simulink model "my_foc9"  (R2024b)
settings: Solver=FixedStepDiscrete  StartTime=0.0  StopTime=2  FixedStep=0.000001  RelTol=1e-3  EnableMultiTasking=on
InitFcn:
  | D_PI_P = 2.19
  | D_PI_I = 1650.0
  | D_PI_UP_LIMIT = 3.0
  | D_PI_LOW_LIMIT = -3.0
  | D_PI_KB = 15
  | 
  | Q_PI_P = 2.19
  | Q_PI_I = 1650.0
  | Q_PI_UP_LIMIT = 3.0
  | Q_PI_LOW_LIMIT = -3.0
  | Q_PI_KB = 15
  | 
  | R = 0.6
  | Ld = 0.000558
  | Lq = 0.000558
  | Pn = 4
  | flux = 0.00572
  | PI = 3.1415926
  | Ts = 0.0001
values from neighbouring files (symbols this model uses):
  D_Upper_lower : value not decoded    [My_PID_parameter.sldd]
  OUT_limits : value not decoded    [My_PID_parameter.sldd]
  Q_KI = 1650.0    [My_PID_parameter.sldd]
  Q_KP = 2.19    [My_PID_parameter.sldd]
  SPEED_PI_I = 3.0    [My_PID_parameter.sldd]
  SPEED_PI_KB = 0.15    [My_PID_parameter.sldd]
  SPEED_PI_LOW_LIMIT = -5.0    [My_PID_parameter.sldd]
  SPEED_PI_P = 0.02    [My_PID_parameter.sldd]
  SPEED_PI_UP_LIMIT = 5.0    [My_PID_parameter.sldd]
undefined symbols (not defined in the file or in its folder): DiscIntNeverNeededParam
libraries: slpidlib x2, spsDCVoltageSourceLib x1, spsGroundLib x1, spsPermanentMagnetSynchronousMachineLib x1, simulink x1, spsThreePhaseVIMeasurementLib x1, spsUniversalBridgeLib x1, spspowerguiLib x1
settings Model: DataDictionary=My_PID_parameter.sldd  EnableAccessToBaseWorkspace=off  Creator=HRT  LastModifiedBy=12894
settings SolverCC: AlgebraicLoopSolver=TrustRegion
settings DataIOCC: ReturnWorkspaceOutputs=off
settings OptimizationCC: DefaultParameterBehavior=Inlined  UseDivisionForNetSlopeComputation=on  UseFloatMulNetSlope=on  DefaultUnderspecifiedDataType=single  InlineInvariantSignals=on  PassReuseOutputArgsAs=Individual arguments  ZeroExternalMemoryAtStartup=off  ZeroInternalMemoryAtStartup=off  NoFixptDivByZeroProtection=on  EfficientFloat2IntCast=on  LifeSpan=1  MaxStackSize=64  OptimizeBlockOrder=speed  DifferentSizesBufferReuse=on  EfficientTunableParamExpr=on
settings DebuggingCC: ParameterTunabilityLossMsg=error  UnconnectedInputMsg=warning  UnconnectedOutputMsg=warning  UnconnectedLineMsg=warning  ArithmeticOperatorsInVariantConditions=warning
settings HardwareCC: ProdBitPerPointer=32  ProdBitPerSizeT=32  ProdBitPerPtrDiffT=32  ProdLargestAtomicInteger=Long  ProdLargestAtomicFloat=Double  ProdWordSize=32  ProdLongLongMode=on  ProdHWDeviceType=ARM Compatible->ARM Cortex
settings ModelReferenceCC: EnableRefExpFcnMdlSchedulingChecks=on
settings SFSimCC: MATLABDynamicMemAlloc=off  CustomCodeUndefinedFunction=UseInterfaceOnly
settings RTWCC: Description=Embedded Coder  SystemTargetFile=ert.tlc  HardwareBoard=STM32F4-Discovery  TemplateMakefile=ert_default_tmf  GenerateReport=on  Toolchain=GNU Tools for ARM Embedded Processors  IncludeHyperlinkInReport=on  LaunchReport=on  GenerateTraceInfo=on  GenerateTraceReport=on  GenerateTraceReportSl=on  GenerateTraceReportSf=on  GenerateTraceReportEml=on  GenerateCodeMetricsReport=on  GPUComputeCapability=3.5
settings CodeAppCC: ForceParamTrailComments=on  IgnoreCustomStorageClasses=off  OperatorAnnotations=on  SimulinkDataObjDesc=on  SFDataObjDesc=on  CustomSymbolStrGlobalVar=rt$N$M  CustomSymbolStrType=$N$M  CustomSymbolStrFcn=$N$M$F  CustomSymbolStrMacro=$N$M  InsertBlockDesc=on
settings ERTTargetCC: CodeReplacementLibrary=ARM Cortex-M (CMSIS)  IncludeMdlTerminateFcn=off  CombineSignalStateStructs=on  SupportComplex=off  SupportNonInlinedSFcns=on  ERTFilePackagingFormat=CompactWithDataFile  DynamicArrayContainerType=coder::array

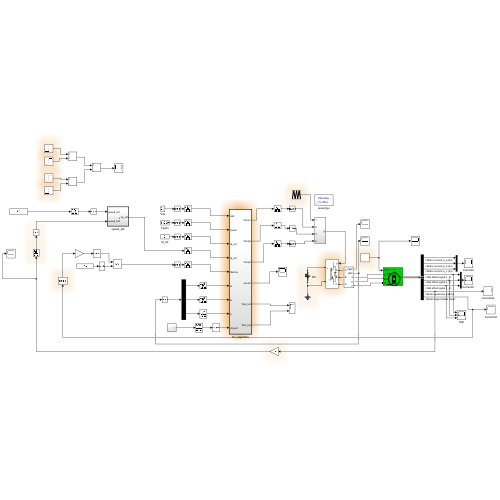
[thumbnail: Simulink's stored preview of the top-level diagram]
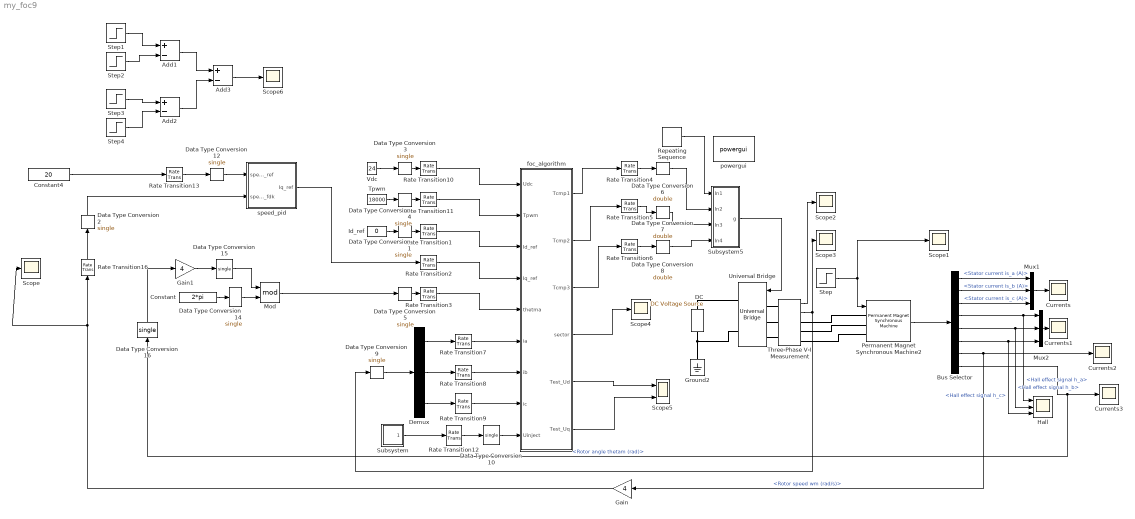
== system my_foc9 ==
  Add1 : Sum  Inputs=+-
  Add2 : Sum  Inputs=+-
  Add3 : Sum  Inputs=+-
  Bus Selector : BusSelector  OutputSignals=Stator current is_a (A),Stator current is_b (A),Stator current is_c (A),Hall effect signal h_a,Hall effect signal h_b,Hall effect signal h_c,Rotor speed wm (rad/s),Rotor angle thetam (rad)
  Constant : Constant  Value=2*pi
  Constant4 : Constant  Value=20  OutDataTypeStr=single
  Currents{,1..3} (4 alike) : Scope
  "DC " : spsDCVoltageSourceLib/DC Voltage Source  Amplitude=24  Measurements=None
  Data Type Conversion{1..5,9..10,12,14..16} (11 alike) : DataTypeConversion  OutDataTypeStr=single  SaturateOnIntegerOverflow=off  RndMeth=Floor
  Data Type Conversion6 : DataTypeConversion  OutDataTypeStr=double  SaturateOnIntegerOverflow=off  RndMeth=Floor
  Data Type Conversion7 : DataTypeConversion  OutDataTypeStr=double  SaturateOnIntegerOverflow=off  RndMeth=Floor
  Data Type Conversion8 : DataTypeConversion  OutDataTypeStr=double  SaturateOnIntegerOverflow=off  RndMeth=Floor
  Demux : Demux  Outputs=3
  Gain : Gain  Gain=4
  Gain1 : Gain  Gain=4
  Ground2 : spsGroundLib/Ground  LConnTagsString=a
  Hall : Scope  NumInputPorts=3
  Id_ref : Constant  Value=0
  Mod : Math  Operator=mod  SignedPower=on
  Mux1 : Mux  Inputs=3
  Mux2 : Mux  Inputs=3
  Permanent Magnet Synchronous Machine2 : spsPermanentMagnetSynchronousMachineLib/Permanent Magnet Synchronous Machine  NbPhases=3  FluxDistribution=Sinusoidal  RotorType=Round  MechanicalLoad=Torque Tm  PresetModel=No  ShowDetailedParameters=on  MeasurementBus=off  Resistance=0.6  Inductance=8.5e-3  dqInductances=[8.5e-3, 8.5e-3]  La=5.58e-4  MachineConstant=Flux linkage established by magnets (V.s)  Flux=0.00572  VoltageCst=4.15  TorqueCst=0.03432  Flat=120  Mechanical=[1.1e-5,1e-4,4,0.02]  PolePairs=4  InitialConditions=[0,0, 0,0]  InitialConditions5ph=[0 0 0 0 0 0]  RefAngle=Aligned with phase A axis (original Park)  IterativeDiscreteModel=Trapezoidal non iterative  TsBlock=-1  TsPowergui=0
  Rate Transition{1..13,16} (14 alike) : RateTransition
  Repeating Sequence : simulink/Sources/Repeating Sequence  rep_seq_t=[0 0.0001 0.0002]  rep_seq_y=[0 9000 0]
  Scope{,1..4,6} (6 alike) : Scope
  Scope5 : Scope  NumInputPorts=2
  Step : Step  Time=0  After=0  SampleTime=0
  Step1 : Step  Time=0.1  After=2  SampleTime=0
  Step2 : Step  Time=0.11  After=2  SampleTime=0
  Step3 : Step  Time=0.13  After=2  SampleTime=0
  Step4 : Step  Time=0.14  After=2  SampleTime=0
  Subsystem : Subsystem
  Subsystem5 : Subsystem
  Three-Phase V-I Measurement : spsThreePhaseVIMeasurementLib/Three-Phase V-I Measurement  VoltageMeasurement=phase-to-ground  SetLabelV=off  LabelV=Vabc  Vpu=off  VpuLL=off  CurrentMeasurement=yes  SetLabelI=off  LabelI=Iabc  Ipu=off  Pbase=100e6  Vbase=500e3  OutputType=Complex  PhasorSimulation=off  PSBequivalent=0
  Tpwm : Constant  Value=18000
  Universal Bridge : spsUniversalBridgeLib/Universal Bridge  Arms=3  SnubberResistance=1e5  SnubberCapacitance=inf  Device=IGBT / Diodes  Ron=1e-3  Lon=0  ForwardVoltages="[  0  0  ]"  ForwardVoltage=0  GTOparameters=[ 10e-6 , 20e-6 ]  IGBTparameters=[ 1e-6 , 2e-6 ]  Measurements=None  Measurements_2=None  converterType=Rectifier
  Vdc : Constant  Value=24
  foc_algorithm : Subsystem  TreatAsAtomicUnit=on  SystemSampleTime=0.0001
  powergui : spspowerguiLib/powergui  Priority=1  SimulationMode=Discrete  SampleTime=0.000001  frequency=60  Iterations=50  frequencyindice=0  Pbase=100e6  ErrMax=1e-4  UnitsV=kV  UnitsW=MW  buscounter=0  FunctionMessages=off  echomessages=off  EnableUseOfTLC=off  CurrentSourceSwitches=off  DisableSnubberDevices=off  DisableRonSwitches=off  DisableVfSwitches=off  DisplayEquations=off  AutomaticDiscreteSolvers=off  SolverType=Tustin/Backward Euler (TBE)  Interpol=off  ExternalGateDelay=off  methode=off  Ts=100  x0status=blocks  SPID=off  SwTol=0  HookPort=off  NonlinearTolerance=1e-4  nMaxIteration=100  ContinueOnMaxIteration=off  RestoreLinks=warning  ResistiveCurrentMeasurement=off  Frange=[0:2:500]  Ylog=off  Xlog=on  ShowGrid=off  save=off  variable=ZData  structure=0  ZoomFFT=off  StartTime=0.0  cycles=1  DisplayStyle=1  fundamental=60  FreqAxis=off  MaxFrequency=1000  frequencyindicesteady=1  RmsSteady=1  display=off
  speed_pid : Subsystem  TreatAsAtomicUnit=on  SystemSampleTime=0.001
  wires:
  Mux2/1 -> Currents1/1
  Rate Transition6/1 -> Data Type Conversion8/1
  Rate Transition10/1 -> foc_algorithm/1(Udc)
  Vdc/1 -> Data Type Conversion3/1
  Data Type Conversion8/1 -> Subsystem5/4(In4)
  Bus Selector/4 -> Hall/1, Mux2/1  "<Hall effect signal h_a>"
  Id_ref/1 -> Data Type Conversion1/1
  Rate Transition2/1 -> foc_algorithm/4(Iq_ref)
  Rate Transition3/1 -> foc_algorithm/5(thetma)
  Mux1/1 -> Currents/1
  Three-Phase V-I Measurement/1 -> Scope2/1
  Data Type Conversion1/1 -> Rate Transition1/1
  Bus Selector/6 -> Mux2/3, Hall/3  "<Hall effect signal h_c>"
  Bus Selector/2 -> Mux1/2  "<Stator current is_b (A)>"
  Bus Selector/7 -> Gain/1, Currents2/1  "<Rotor speed wm (rad/s)>"
  Rate Transition5/1 -> Data Type Conversion7/1
  Rate Transition1/1 -> foc_algorithm/3(Id_ref)
  Data Type Conversion7/1 -> Subsystem5/3(In3)
  Repeating Sequence/1 -> Subsystem5/1(In1)
  foc_algorithm/1(Tcmp1) -> Rate Transition4/1
  Bus Selector/5 -> Mux2/2, Hall/2  "<Hall effect signal h_b>"
  foc_algorithm/3(Tcmp3) -> Rate Transition6/1
  Data Type Conversion5/1 -> Rate Transition3/1
  Rate Transition11/1 -> foc_algorithm/2(Tpwm)
  Bus Selector/3 -> Mux1/3  "<Stator current is_c (A)>"
  foc_algorithm/2(Tcmp2) -> Rate Transition5/1
  Data Type Conversion4/1 -> Rate Transition11/1
  Rate Transition4/1 -> Data Type Conversion6/1
  Data Type Conversion3/1 -> Rate Transition10/1
  Tpwm/1 -> Data Type Conversion4/1
  Bus Selector/8 -> Data Type Conversion16/1, Currents3/1  "<Rotor angle thetam (rad)>"
  Data Type Conversion6/1 -> Subsystem5/2(In2)
  Subsystem5/1(g) -> Universal Bridge/1
  speed_pid/1(Iq_ref) -> Rate Transition2/1
  Bus Selector/1 -> Mux1/1  "<Stator current is_a (A)>"
  foc_algorithm/4(sector) -> Scope4/1
  Demux/3 -> Rate Transition9/1
  Three-Phase V-I Measurement/2 -> Scope3/1, Data Type Conversion9/1
  Demux/2 -> Rate Transition8/1
  Demux/1 -> Rate Transition7/1
  Rate Transition7/1 -> foc_algorithm/6(ia)
  Rate Transition8/1 -> foc_algorithm/7(ib)
  Rate Transition9/1 -> foc_algorithm/8(ic)
  Data Type Conversion9/1 -> Demux/1
  Step/1 -> Permanent Magnet Synchronous Machine2/1, Scope1/1
  foc_algorithm/5(Test_Ud) -> Scope5/1
  foc_algorithm/6(Test_Uq) -> Scope5/2
  Gain1/1 -> Data Type Conversion15/1
  Rate Transition13/1 -> Data Type Conversion12/1
  Constant/1 -> Data Type Conversion14/1
  Data Type Conversion14/1 -> Mod/2
  Data Type Conversion16/1 -> Gain1/1
  Permanent Magnet Synchronous Machine2/1 -> Bus Selector/1
  Data Type Conversion15/1 -> Mod/1
  Constant4/1 -> Rate Transition13/1
  Rate Transition16/1 -> Data Type Conversion2/1
  Data Type Conversion2/1 -> speed_pid/2(speed_fdk)
  Gain/1 -> Scope/1, Rate Transition16/1
  Mod/1 -> Data Type Conversion5/1
  Step1/1 -> Add1/1
  Step2/1 -> Add1/2
  Step3/1 -> Add2/1
  Step4/1 -> Add2/2
  Add1/1 -> Add3/1
  Add2/1 -> Add3/2
  Add3/1 -> Scope6/1
  Subsystem/1(Out1) -> Rate Transition12/1
  Rate Transition12/1 -> Data Type Conversion10/1
  Data Type Conversion10/1 -> foc_algorithm/9("Uinject ")
  Data Type Conversion12/1 -> speed_pid/1(speed_ref)
  connections:
  Ground2/LConn1 -- Universal Bridge/RConn2 -- "DC "/LConn1
  "DC "/RConn1 -- Universal Bridge/RConn1
  Universal Bridge/LConn2 -- Three-Phase V-I Measurement/LConn2
  Universal Bridge/LConn1 -- Three-Phase V-I Measurement/LConn1
  Permanent Magnet Synchronous Machine2/LConn3 -- Three-Phase V-I Measurement/RConn3
  Universal Bridge/LConn3 -- Three-Phase V-I Measurement/LConn3
  Permanent Magnet Synchronous Machine2/LConn2 -- Three-Phase V-I Measurement/RConn2
  Permanent Magnet Synchronous Machine2/LConn1 -- Three-Phase V-I Measurement/RConn1

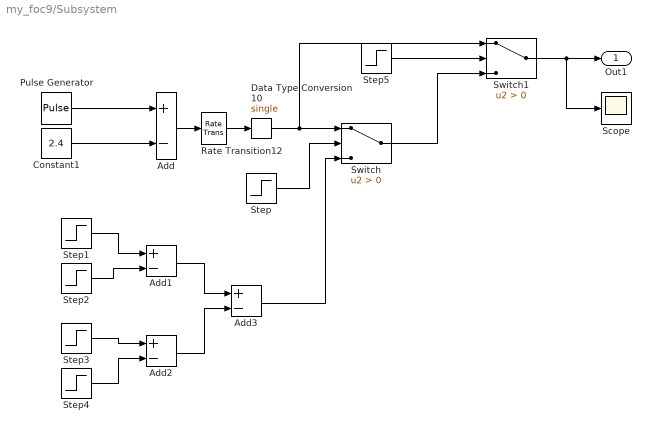
== system my_foc9/Subsystem ==
  Add{,1..3} (4 alike) : Sum  Inputs=+-
  Constant1 : Constant  Value=2.4
  Data Type Conversion10 : DataTypeConversion  OutDataTypeStr=single  SaturateOnIntegerOverflow=off  RndMeth=Floor
  Pulse Generator : DiscretePulseGenerator  PulseType=Time based  Amplitude=4.8  Period=0.0002  PulseWidth=50
  Rate Transition12 : RateTransition
  Scope : Scope
  Step : Step  Time=0.5  Before=1  After=0  SampleTime=0
  Step1 : Step  Time=0.6  After=2  SampleTime=0
  Step2 : Step  Time=0.7  After=2  SampleTime=0
  Step3 : Step  Time=0.8  After=2  SampleTime=0
  Step4 : Step  Time=0.9  After=2  SampleTime=0
  Step5 : Step  After=2  SampleTime=0
  Switch : Switch  Criteria=u2 > Threshold  SaturateOnIntegerOverflow=off  InputSameDT=off
  Switch1 : Switch  Criteria=u2 > Threshold  SaturateOnIntegerOverflow=off  InputSameDT=off
  Out1 : Outport  VectorParamsAs1DForOutWhenUnconnected=off
  wires:
  Constant1/1 -> Add/2
  Rate Transition12/1 -> Data Type Conversion10/1
  Pulse Generator/1 -> Add/1
  Add/1 -> Rate Transition12/1
  Switch/1 -> Switch1/3
  Step3/1 -> Add2/1
  Step1/1 -> Add1/1
  Add2/1 -> Add3/2
  Add1/1 -> Add3/1
  Step2/1 -> Add1/2
  Step4/1 -> Add2/2
  Data Type Conversion10/1 -> Switch1/1, Switch/1
  Step/1 -> Switch/2
  Step5/1 -> Switch1/2
  Switch1/1 -> Scope/1, Out1/1
  Add3/1 -> Switch/3

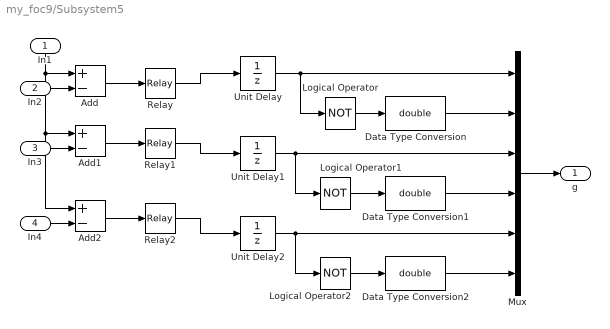
== system my_foc9/Subsystem5 ==
  In1 : Inport
  In2 : Inport  Port=2
  In3 : Inport  Port=3
  In4 : Inport  Port=4
  Add : Sum  Inputs=+-
  Add1 : Sum  Inputs=+-
  Add2 : Sum  Inputs=+-
  Data Type Conversion : DataTypeConversion  OutDataTypeStr=double  SaturateOnIntegerOverflow=off  RndMeth=Floor
  Data Type Conversion1 : DataTypeConversion  OutDataTypeStr=double  SaturateOnIntegerOverflow=off  RndMeth=Floor
  Data Type Conversion2 : DataTypeConversion  OutDataTypeStr=double  SaturateOnIntegerOverflow=off  RndMeth=Floor
  Logical Operator : Logic  Operator=NOT  AllPortsSameDT=off  OutDataTypeStr=boolean
  Logical Operator1 : Logic  Operator=NOT  AllPortsSameDT=off  OutDataTypeStr=boolean
  Logical Operator2 : Logic  Operator=NOT  AllPortsSameDT=off  OutDataTypeStr=boolean
  Mux : Mux  Inputs=6
  Relay : Relay  OffSwitchValue=-eps
  Relay1 : Relay  OffSwitchValue=-eps
  Relay2 : Relay  OffSwitchValue=-eps
  Unit Delay : UnitDelay  SampleTime=-1  HasFrameUpgradeWarning=on
  Unit Delay1 : UnitDelay  SampleTime=-1  HasFrameUpgradeWarning=on
  Unit Delay2 : UnitDelay  SampleTime=-1  HasFrameUpgradeWarning=on
  g : Outport  VectorParamsAs1DForOutWhenUnconnected=off
  wires:
  In4/1 -> Add2/2
  In3/1 -> Add1/2
  In2/1 -> Add/2
  Relay2/1 -> Unit Delay2/1
  Relay1/1 -> Unit Delay1/1
  Relay/1 -> Unit Delay/1
  Unit Delay2/1 -> Mux/5, Logical Operator2/1
  Unit Delay1/1 -> Mux/3, Logical Operator1/1
  Unit Delay/1 -> Logical Operator/1, Mux/1
  Mux/1 -> g/1
  Data Type Conversion/1 -> Mux/2
  Data Type Conversion1/1 -> Mux/4
  Data Type Conversion2/1 -> Mux/6
  Logical Operator2/1 -> Data Type Conversion2/1
  Logical Operator1/1 -> Data Type Conversion1/1
  Logical Operator/1 -> Data Type Conversion/1
  Add1/1 -> Relay1/1
  Add2/1 -> Relay2/1
  Add/1 -> Relay/1
  In1/1 -> Add/1, Add2/1, Add1/1

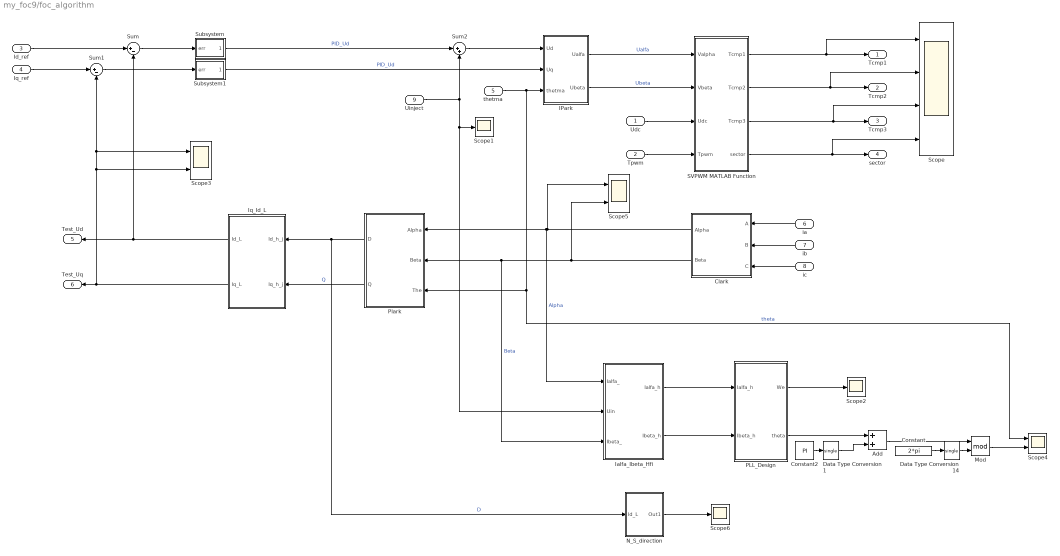
== system my_foc9/foc_algorithm ==
  Udc : Inport
  Tpwm : Inport  Port=2
  Id_ref : Inport  Port=3
  Iq_ref : Inport  Port=4
  thetma : Inport  Port=5
  ia : Inport  Port=6
  ib : Inport  Port=7
  ic : Inport  Port=8
  "Uinject " : Inport  Port=9
  Add : Sum
  Clark : Subsystem
  Constant : Constant  Value=2*pi
  Constant2 : Constant  Value=PI
  Data Type Conversion1 : DataTypeConversion  OutDataTypeStr=single  SaturateOnIntegerOverflow=off  RndMeth=Floor
  Data Type Conversion14 : DataTypeConversion  OutDataTypeStr=single  SaturateOnIntegerOverflow=off  RndMeth=Floor
  IPark : Subsystem
  "Ialfa_Ibeta_Hfi " : Subsystem  TreatAsAtomicUnit=on  SystemSampleTime=Ts
  Iq_Id_L : Subsystem
  Mod : Math  Operator=mod  SignedPower=on
  N_S_direction : Subsystem  TreatAsAtomicUnit=on  SystemSampleTime=Ts
  PLL_Design : Subsystem  TreatAsAtomicUnit=on  SystemSampleTime=Ts
  Plark : Subsystem
  SVPWM MATLAB Function : MATLAB Function  TreatAsAtomicUnit=on
  Scope : Scope  NumInputPorts=4
  Scope1 : Scope
  Scope2 : Scope
  Scope3 : Scope  NumInputPorts=2
  Scope4 : Scope  NumInputPorts=2
  Scope5 : Scope  NumInputPorts=2
  Scope6 : Scope
  Subsystem : Subsystem  mask(my_pi){kp=Q_KP, ki=Q_KI, Intergral_Limits=D_Upper_lower, Output_Limits=OUT_limits, init=0, TS=0.0001}
      mask prompts: kp "Proportional gain(kp):"; ki "Intergral gain(ki):"; Intergral_Limits "Intergral limits:[Upper Lowers]"; Output_Limits "Output limits:[Upper Lower]"; init "Output init value:"; TS "Sample time:"
      mask init:
      | Intergral_upper =Intergral_Limits(1);
      | Intergral_lower = Intergral_Limits(2);
      | Out_upper       = Output_Limits(1);
      | Out_lower       = Output_Limits(2);
      mask Display: disp('PI')
  Subsystem1 : Subsystem  mask(my_pi){kp=Q_KP, ki=Q_KI, Intergral_Limits=D_Upper_lower, Output_Limits=OUT_limits, init=0, TS=0.0001}
      mask prompts: kp "Proportional gain(kp):"; ki "Intergral gain(ki):"; Intergral_Limits "Intergral limits:[Upper Lowers]"; Output_Limits "Output limits:[Upper Lower]"; init "Output init value:"; TS "Sample time:"
      mask init:
      | Intergral_upper =Intergral_Limits(1);
      | Intergral_lower = Intergral_Limits(2);
      | Out_upper       = Output_Limits(1);
      | Out_lower       = Output_Limits(2);
      mask Display: disp('PI')
  Sum : Sum  Inputs=|+-
  Sum1 : Sum  Inputs=|+-
  Sum2 : Sum  Inputs=|++
  Tcmp1 : Outport  VectorParamsAs1DForOutWhenUnconnected=off
  Tcmp2 : Outport  Port=2  VectorParamsAs1DForOutWhenUnconnected=off
  Tcmp3 : Outport  Port=3  VectorParamsAs1DForOutWhenUnconnected=off
  sector : Outport  Port=4  VectorParamsAs1DForOutWhenUnconnected=off
  Test_Ud : Outport  Port=5  VectorParamsAs1DForOutWhenUnconnected=off
  Test_Uq : Outport  Port=6  VectorParamsAs1DForOutWhenUnconnected=off
  wires:
  IPark/1(Ualfa) -> SVPWM MATLAB Function/1(Valpha)  "Ualfa"
  IPark/2(Ubeta) -> SVPWM MATLAB Function/2(Vbeta)  "Ubeta"
  Udc/1 -> SVPWM MATLAB Function/3(Udc)
  Tpwm/1 -> SVPWM MATLAB Function/4(Tpwm)
  SVPWM MATLAB Function/1(Tcmp1) -> Scope/1, Tcmp1/1
  SVPWM MATLAB Function/2(Tcmp2) -> Scope/2, Tcmp2/1
  SVPWM MATLAB Function/3(Tcmp3) -> Scope/3, Tcmp3/1
  thetma/1 -> Scope4/1, Plark/3(The), IPark/3(thetma)  "theta"
  SVPWM MATLAB Function/4(sector) -> Scope/4, sector/1
  Clark/1(Alpha) -> "Ialfa_Ibeta_Hfi "/1(Ialfa_), Plark/1(Alpha), Scope5/1  "Alpha"
  Clark/2(Beta) -> Scope5/2, "Ialfa_Ibeta_Hfi "/3(Ibeta_), Plark/2(Beta)  "Beta"
  Sum/1 -> Subsystem/1("err ")
  Sum1/1 -> Subsystem1/1("err ")
  Plark/1(D) -> N_S_direction/1(Id_L), Iq_Id_L/1(Id_h_j)  "D"
  Plark/2(Q) -> Iq_Id_L/2(Iq_h_j)  "Q"
  ia/1 -> Clark/1(A)
  ib/1 -> Clark/2(B)
  ic/1 -> Clark/3(C)
  Iq_ref/1 -> Sum1/1
  Id_ref/1 -> Sum/1
  "Uinject "/1 -> "Ialfa_Ibeta_Hfi "/2("Uin "), Scope1/1, Sum2/2
  "Ialfa_Ibeta_Hfi "/2(Ibeta_h) -> PLL_Design/2("Ibeta_h ")
  "Ialfa_Ibeta_Hfi "/1("Ialfa_h ") -> PLL_Design/1(Ialfa_h)
  PLL_Design/1("We ") -> Scope2/1
  Sum2/1 -> IPark/1(Ud)
  Subsystem/1(Out1) -> Sum2/1  "PID_Ud"
  Subsystem1/1(Out1) -> IPark/2(Uq)  "PID_Ud"
  Iq_Id_L/2(Iq_L) -> Scope3/2, Sum1/2, Scope3/1, Test_Uq/1
  Iq_Id_L/1(Id_L) -> Sum/2, Test_Ud/1
  Data Type Conversion14/1 -> Mod/2
  Constant/1 -> Data Type Conversion14/1
  Mod/1 -> Scope4/2
  PLL_Design/2(theta) -> Add/1
  Add/1 -> Mod/1
  Constant2/1 -> Data Type Conversion1/1
  Data Type Conversion1/1 -> Add/2
  N_S_direction/1(Out1) -> Scope6/1

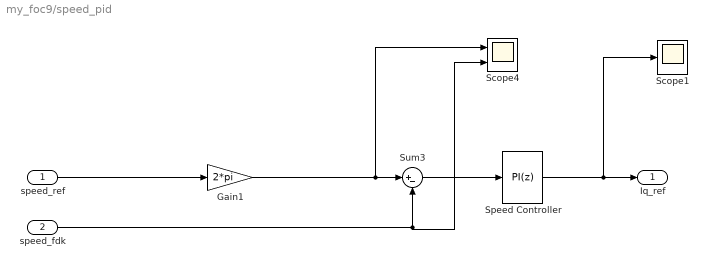
== system my_foc9/speed_pid ==
  speed_ref : Inport
  speed_fdk : Inport  Port=2
  Gain1 : Gain  Gain=2*pi  OutDataTypeStr=single
  Scope1 : Scope
  Scope4 : Scope  NumInputPorts=2
  Speed Controller : slpidlib/PID Controller  Controller=PI  Form=Ideal  TimeDomain=Discrete-time  UseExternalTs=off  SampleTime=-1  IntegratorMethod=Forward Euler  FilterMethod=Forward Euler  ControllerParametersSource=internal  P=SPEED_PI_P  I=SPEED_PI_I  UseKiTs=off  D=0.0005  UseExternalDerivativeSource=off  N=100  UseFilter=on  TunerSelectOption=Transfer Function Based (PID Tuner App)  InitialConditionSource=internal  InitialConditionForIntegrator=0  InitialConditionForFilter=0  DifferentiatorICPrevScaledInput=0  ExternalReset=none  TrackingMode=off  Kt=1  LimitOutput=on  SatLimitsSource=internal  UpperSaturationLimit=SPEED_PI_UP_LIMIT  LowerSaturationLimit=SPEED_PI_LOW_LIMIT  LinearizeAsGain=off  AntiWindupMode=back-calculation  Kb=SPEED_PI_KB  LimitIntegrator=off  UpperIntegratorSaturationLimit=inf  LowerIntegratorSaturationLimit=-inf  PGainOutDataTypeStr=single  PProdOutDataTypeStr=single  POutMin=[]  POutMax=[]  IGainOutDataTypeStr=single  IProdOutDataTypeStr=single  IOutMin=[]  IOutMax=[]  DOutMin=[]  DOutMax=[]  NOutMin=[]  NOutMax=[]  SumOutDataTypeStr=single  SumOutMin=[]  SumOutMax=[]  SaturationOutDataTypeStr=single  SaturationOutMin=[]  SaturationOutMax=[]  PParamDataTypeStr=single  PParamMin=[]  PParamMax=[]  IParamDataTypeStr=single  IParamMin=[]  IParamMax=[]  DParamMin=[]  DParamMax=[]  NParamMin=[]  NParamMax=[]  KbParamDataTypeStr=single  KbParamMin=[]  KbParamMax=[]  KtParamMin=[]  KtParamMax=[]  KbOutDataTypeStr=single  KbOutMin=[]  KbOutMax=[]  KtOutMin=[]  KtOutMax=[]  IntegratorOutDataTypeStr=single  IntegratorOutMin=[]  IntegratorOutMax=[]  FilterOutMin=[]  FilterOutMax=[]  SumI1OutDataTypeStr=single  SumI1OutMin=[]  SumI1OutMax=[]  SumI2OutDataTypeStr=single  SumI2OutMin=[]  SumI2OutMax=[]  SumI3OutMin=[]  SumI3OutMax=[]  SumI4OutMin=[]  SumI4OutMax=[]  SumDOutMin=[]  SumDOutMax=[]  SumAccumDataTypeStr=single  SumI1AccumDataTypeStr=single  SumI2AccumDataTypeStr=single  DifferentiatorOutMin=[]  DifferentiatorOutMax=[]  FilterDiffOutCoefMin=[]  FilterDiffOutCoefMax=[]  ReciprocalOutMin=[]  ReciprocalOutMax=[]  SumDenOutMin=[]  SumDenOutMax=[]  SumNumOutMin=[]  SumNumOutMax=[]  DivideOutMin=[]  DivideOutMax=[]  UdiffTsProdOutMin=[]  UdiffTsProdOutMax=[]  NTsProdOutMin=[]  NTsProdOutMax=[]  UintegralTsProdOutMin=[]  UintegralTsProdOutMax=[]  UngainTsProdOutMin=[]  UngainTsProdOutMax=[]  ClampingZeroOutDataTypeStr=Inherit: Inherit via back propagation  ClampingZeroOutMin=[]  ClampingZeroOutMax=[]  FilterDenConstantOutDataTypeStr=Inherit: Inherit via back propagation  FilterDenConstantOutMin=[]  FilterDenConstantOutMax=[]  PCopyOutDataTypeStr=Inherit: Inherit via back propagation  PCopyOutMin=[]  PCopyOutMax=[]  NCopyOutDataTypeStr=Inherit: Inherit via back propagation  NCopyOutMin=[]  NCopyOutMax=[]  IntegratorContinuousStateAttributes=''  IntegratorStateIdentifier=si  IntegratorStateMustResolveToSignalObject=off  IntegratorRTWStateStorageClass=Auto  FilterContinuousStateAttributes=''  FilterStateMustResolveToSignalObject=off  FilterRTWStateStorageClass=Auto  ParallelPVariant=Passthrough  IdealPVariant=InternalParameters  IVariant=InternalParameters  DVariant=Disabled  IntegratorVariant=Discrete  SatVariant=Enabled  AWVariant=BackCalculation  PCopyVariant=Disabled  TRVariant=Disabled  FdbkBlocksVariant=Forward  IdealPFdbkVariant=Disabled  SatFdbkVariant=Disabled  DerivativeFilterVariant=Disabled  NVariant=Disabled  NCopyVariant=Disabled_SignalSpec  FilterICVariant=Disabled  IntegratorICVariant=InternalICs  ExternalResetVariant=Disabled  TRSumVariant=Passthrough  SumFdbkVariant=Disabled  SumVariant=Sum_PI  TsampFilterVariant=InternalTs  TsampNgainVariant=Passthrough  TsampIntegralVariant=Disabled_SignalSpec  ExternalSaturationOutDataTypeStr=Inherit: Same as second input  DerivativeSourceVariant=Disabled  PreIntVariant=InternalPreInt
  Sum3 : Sum  Inputs=|+-  InputSameDT=on
  Iq_ref : Outport  VectorParamsAs1DForOutWhenUnconnected=off
  wires:
  Sum3/1 -> Speed Controller/1
  speed_ref/1 -> Gain1/1
  Speed Controller/1 -> Scope1/1, Iq_ref/1
  speed_fdk/1 -> Scope4/2, Sum3/2
  Gain1/1 -> Sum3/1, Scope4/1

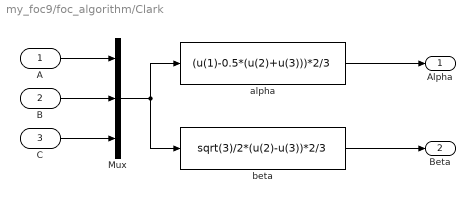
== system my_foc9/foc_algorithm/Clark ==
  A : Inport
  B : Inport  Port=2
  C : Inport  Port=3
  Mux : Mux  Inputs=3
  alpha : Fcn  Expr=(u(1)-0.5*(u(2)+u(3)))*2/3
  beta : Fcn  Expr=sqrt(3)/2*(u(2)-u(3))*2/3
  Alpha : Outport  VectorParamsAs1DForOutWhenUnconnected=off
  Beta : Outport  Port=2  VectorParamsAs1DForOutWhenUnconnected=off
  wires:
  alpha/1 -> Alpha/1
  B/1 -> Mux/2
  C/1 -> Mux/3
  A/1 -> Mux/1
  Mux/1 -> beta/1, alpha/1
  beta/1 -> Beta/1

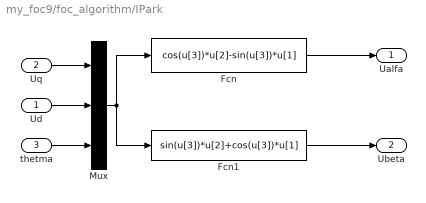
== system my_foc9/foc_algorithm/IPark ==
  Ud : Inport
  Uq : Inport  Port=2
  thetma : Inport  Port=3
  Fcn : Fcn  Expr=cos(u[3])*u[2]-sin(u[3])*u[1]
  Fcn1 : Fcn  Expr=sin(u[3])*u[2]+cos(u[3])*u[1]
  Mux : Mux  Inputs=3
  Ualfa : Outport  VectorParamsAs1DForOutWhenUnconnected=off
  Ubeta : Outport  Port=2  VectorParamsAs1DForOutWhenUnconnected=off
  wires:
  Uq/1 -> Mux/1
  Ud/1 -> Mux/2
  thetma/1 -> Mux/3
  Mux/1 -> Fcn/1, Fcn1/1
  Fcn/1 -> Ualfa/1
  Fcn1/1 -> Ubeta/1

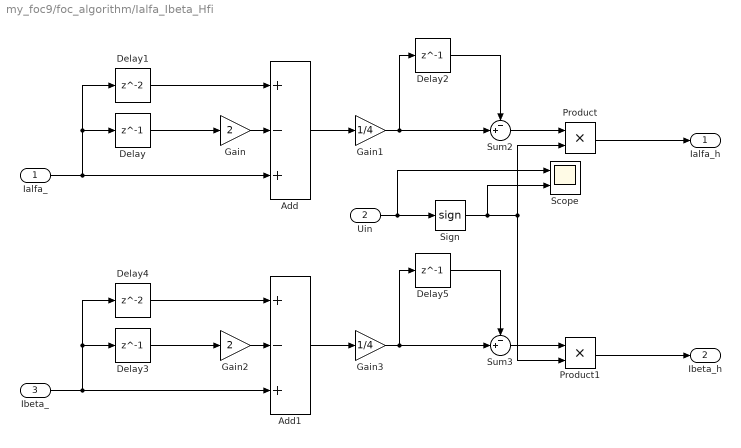
== system my_foc9/foc_algorithm/Ialfa_Ibeta_Hfi  ==
  Ialfa_ : Inport
  "Uin " : Inport  Port=2
  Ibeta_ : Inport  Port=3
  Add : Sum  Inputs=+-+
  Add1 : Sum  Inputs=+-+
  Delay{,2..3,5} (4 alike) : Delay  DelayLength=1  SampleTime=Ts
  Delay1 : Delay  SampleTime=Ts
  Delay4 : Delay  SampleTime=Ts
  Gain : Gain  Gain=2
  Gain1 : Gain  Gain=1/4
  Gain2 : Gain  Gain=2
  Gain3 : Gain  Gain=1/4
  Product : Product
  Product1 : Product
  Scope : Scope  NumInputPorts=2
  Sign : Signum
  Sum2 : Sum  Inputs=-+|
  Sum3 : Sum  Inputs=-+|
  "Ialfa_h " : Outport  VectorParamsAs1DForOutWhenUnconnected=off
  Ibeta_h : Outport  Port=2  VectorParamsAs1DForOutWhenUnconnected=off
  wires:
  Sign/1 -> Scope/2, Product/2, Product1/2
  Ialfa_/1 -> Delay1/1, Delay/1, Add/3
  "Uin "/1 -> Scope/1, Sign/1
  Gain3/1 -> Delay5/1, Sum3/2
  Ibeta_/1 -> Delay4/1, Delay3/1, Add1/3
  Gain/1 -> Add/2
  Gain1/1 -> Delay2/1, Sum2/2
  Delay1/1 -> Add/1
  Gain2/1 -> Add1/2
  Sum2/1 -> Product/1
  Add1/1 -> Gain3/1
  Sum3/1 -> Product1/1
  Product1/1 -> Ibeta_h/1
  Delay5/1 -> Sum3/1
  Delay3/1 -> Gain2/1
  Product/1 -> "Ialfa_h "/1
  Delay4/1 -> Add1/1
  Delay2/1 -> Sum2/1
  Delay/1 -> Gain/1
  Add/1 -> Gain1/1

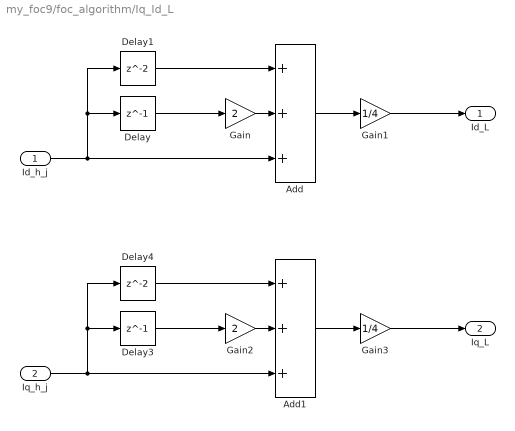
== system my_foc9/foc_algorithm/Iq_Id_L ==
  Id_h_j : Inport
  Iq_h_j : Inport  Port=2
  Add : Sum  Inputs=+++
  Add1 : Sum  Inputs=+++
  Delay : Delay  DelayLength=1  SampleTime=Ts
  Delay1 : Delay  SampleTime=Ts
  Delay3 : Delay  DelayLength=1  SampleTime=Ts
  Delay4 : Delay  SampleTime=Ts
  Gain : Gain  Gain=2
  Gain1 : Gain  Gain=1/4
  Gain2 : Gain  Gain=2
  Gain3 : Gain  Gain=1/4
  Id_L : Outport  VectorParamsAs1DForOutWhenUnconnected=off
  Iq_L : Outport  Port=2  VectorParamsAs1DForOutWhenUnconnected=off
  wires:
  Delay3/1 -> Gain2/1
  Iq_h_j/1 -> Delay4/1, Delay3/1, Add1/3
  Delay1/1 -> Add/1
  Gain/1 -> Add/2
  Gain2/1 -> Add1/2
  Delay4/1 -> Add1/1
  Add/1 -> Gain1/1
  Add1/1 -> Gain3/1
  Delay/1 -> Gain/1
  Id_h_j/1 -> Delay1/1, Delay/1, Add/3
  Gain1/1 -> Id_L/1
  Gain3/1 -> Iq_L/1

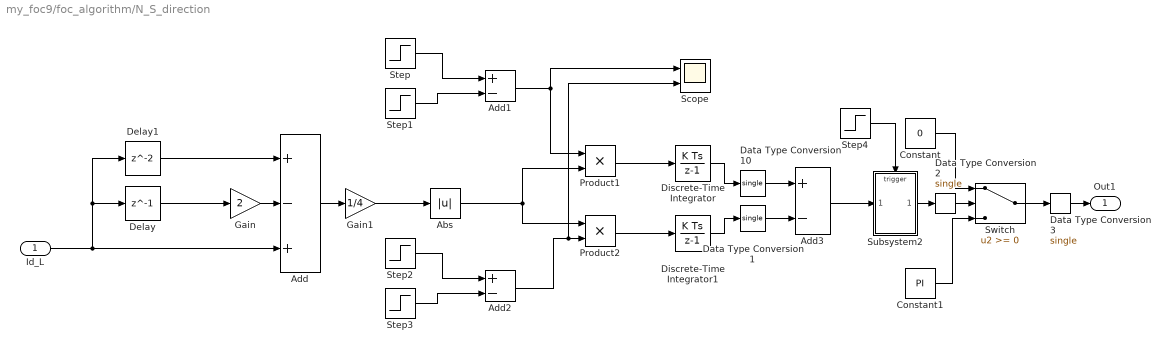
== system my_foc9/foc_algorithm/N_S_direction ==
  Id_L : Inport
  Abs : Abs  SaturateOnIntegerOverflow=off
  Add : Sum  Inputs=+-+
  Add1 : Sum  Inputs=+-
  Add2 : Sum  Inputs=+-
  Add3 : Sum  Inputs=+-
  Constant : Constant  Value=0
  Constant1 : Constant  Value=PI
  Data Type Conversion{1..3,10} (4 alike) : DataTypeConversion  OutDataTypeStr=single  SaturateOnIntegerOverflow=off  RndMeth=Floor
  Delay : Delay  DelayLength=1  SampleTime=Ts
  Delay1 : Delay  SampleTime=Ts
  Discrete-Time Integrator : DiscreteIntegrator  SampleTime=Ts  ICPrevOutput=DiscIntNeverNeededParam  ICPrevScaledInput=DiscIntNeverNeededParam
  Discrete-Time Integrator1 : DiscreteIntegrator  SampleTime=Ts  ICPrevOutput=DiscIntNeverNeededParam  ICPrevScaledInput=DiscIntNeverNeededParam
  Gain : Gain  Gain=2
  Gain1 : Gain  Gain=1/4
  Product1 : Product
  Product2 : Product
  Scope : Scope  NumInputPorts=2
  Step : Step  Time=0.6  After=2  SampleTime=Ts
  Step1 : Step  Time=0.7  After=2  SampleTime=Ts
  Step2 : Step  Time=0.8  After=2  SampleTime=Ts
  Step3 : Step  Time=0.9  After=2  SampleTime=Ts
  Step4 : Step  Time=0.16  SampleTime=Ts
  Subsystem2 : Subsystem
  Switch : Switch  SaturateOnIntegerOverflow=off  InputSameDT=off
  Out1 : Outport  VectorParamsAs1DForOutWhenUnconnected=off
  wires:
  Step4/1 -> Subsystem2/Trigger
  Switch/1 -> Data Type Conversion3/1
  Add2/1 -> Scope/2, Product2/2
  Step/1 -> Add1/1
  Product2/1 -> Discrete-Time Integrator1/1
  Gain/1 -> Add/2
  Delay1/1 -> Add/1
  Step2/1 -> Add2/1
  Product1/1 -> Discrete-Time Integrator/1
  Gain1/1 -> Abs/1
  Constant/1 -> Switch/1
  Id_L/1 -> Delay1/1, Delay/1, Add/3
  Add3/1 -> Subsystem2/1(In1)
  Subsystem2/1(Out1) -> Data Type Conversion2/1
  Step3/1 -> Add2/2
  Add1/1 -> Product1/1, Scope/1
  Abs/1 -> Product2/1, Product1/2
  Delay/1 -> Gain/1
  Add/1 -> Gain1/1
  Step1/1 -> Add1/2
  Constant1/1 -> Switch/3
  Data Type Conversion10/1 -> Add3/1
  Discrete-Time Integrator/1 -> Data Type Conversion10/1
  Data Type Conversion1/1 -> Add3/2
  Discrete-Time Integrator1/1 -> Data Type Conversion1/1
  Data Type Conversion2/1 -> Switch/2
  Data Type Conversion3/1 -> Out1/1

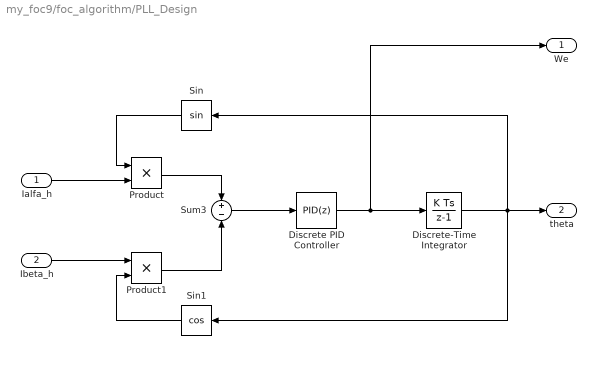
== system my_foc9/foc_algorithm/PLL_Design ==
  Ialfa_h : Inport
  "Ibeta_h " : Inport  Port=2
  Discrete PID Controller : slpidlib/PID Controller  Controller=PID  Form=Parallel  TimeDomain=Discrete-time  UseExternalTs=off  SampleTime=Ts  IntegratorMethod=Forward Euler  FilterMethod=Forward Euler  ControllerParametersSource=internal  P=540  I=8600  UseKiTs=off  D=0  UseExternalDerivativeSource=off  N=100  UseFilter=on  TunerSelectOption=Transfer Function Based (PID Tuner App)  InitialConditionSource=internal  InitialConditionForIntegrator=0  InitialConditionForFilter=0  DifferentiatorICPrevScaledInput=0  ExternalReset=none  TrackingMode=off  Kt=1  LimitOutput=off  SatLimitsSource=internal  UpperSaturationLimit=inf  LowerSaturationLimit=-inf  LinearizeAsGain=off  AntiWindupMode=none  Kb=1  LimitIntegrator=off  UpperIntegratorSaturationLimit=inf  LowerIntegratorSaturationLimit=-inf  POutMin=[]  POutMax=[]  IOutMin=[]  IOutMax=[]  DOutMin=[]  DOutMax=[]  NOutMin=[]  NOutMax=[]  SumOutMin=[]  SumOutMax=[]  SaturationOutMin=[]  SaturationOutMax=[]  PParamMin=[]  PParamMax=[]  IParamMin=[]  IParamMax=[]  DParamMin=[]  DParamMax=[]  NParamMin=[]  NParamMax=[]  KbParamMin=[]  KbParamMax=[]  KtParamMin=[]  KtParamMax=[]  KbOutMin=[]  KbOutMax=[]  KtOutMin=[]  KtOutMax=[]  IntegratorOutMin=[]  IntegratorOutMax=[]  FilterOutMin=[]  FilterOutMax=[]  SumI1OutMin=[]  SumI1OutMax=[]  SumI2OutMin=[]  SumI2OutMax=[]  SumI3OutMin=[]  SumI3OutMax=[]  SumI4OutMin=[]  SumI4OutMax=[]  SumDOutMin=[]  SumDOutMax=[]  DifferentiatorOutMin=[]  DifferentiatorOutMax=[]  FilterDiffOutCoefMin=[]  FilterDiffOutCoefMax=[]  ReciprocalOutMin=[]  ReciprocalOutMax=[]  SumDenOutMin=[]  SumDenOutMax=[]  SumNumOutMin=[]  SumNumOutMax=[]  DivideOutMin=[]  DivideOutMax=[]  UdiffTsProdOutMin=[]  UdiffTsProdOutMax=[]  NTsProdOutMin=[]  NTsProdOutMax=[]  UintegralTsProdOutMin=[]  UintegralTsProdOutMax=[]  UngainTsProdOutMin=[]  UngainTsProdOutMax=[]  ClampingZeroOutDataTypeStr=Inherit: Inherit via back propagation  ClampingZeroOutMin=[]  ClampingZeroOutMax=[]  FilterDenConstantOutDataTypeStr=Inherit: Inherit via back propagation  FilterDenConstantOutMin=[]  FilterDenConstantOutMax=[]  PCopyOutDataTypeStr=Inherit: Inherit via back propagation  PCopyOutMin=[]  PCopyOutMax=[]  NCopyOutDataTypeStr=Inherit: Inherit via back propagation  NCopyOutMin=[]  NCopyOutMax=[]  IntegratorContinuousStateAttributes=''  IntegratorStateMustResolveToSignalObject=off  IntegratorRTWStateStorageClass=Auto  FilterContinuousStateAttributes=''  FilterStateMustResolveToSignalObject=off  FilterRTWStateStorageClass=Auto  ParallelPVariant=InternalParameters  IdealPVariant=Disabled  IVariant=InternalParameters  DVariant=InternalParameters  IntegratorVariant=Discrete  SatVariant=Disabled  AWVariant=Passthrough  PCopyVariant=Disabled  TRVariant=Disabled  FdbkBlocksVariant=Forward  IdealPFdbkVariant=Disabled  SatFdbkVariant=Disabled  DerivativeFilterVariant=ForwardEulerFilter  NVariant=InternalParameters  NCopyVariant=Disabled  FilterICVariant=InternalICsFilter  IntegratorICVariant=InternalICs  ExternalResetVariant=Disabled  TRSumVariant=Passthrough  SumFdbkVariant=Disabled  SumVariant=Sum_PID  TsampFilterVariant=InternalTs  TsampNgainVariant=Passthrough  TsampIntegralVariant=Disabled_SignalSpec  ExternalSaturationOutDataTypeStr=Inherit: Same as second input  DerivativeSourceVariant=ErrorSignal  PreIntVariant=InternalPreInt
  Discrete-Time Integrator : DiscreteIntegrator  SampleTime=-1  ICPrevOutput=DiscIntNeverNeededParam  ICPrevScaledInput=DiscIntNeverNeededParam
  Product : Product
  Product1 : Product
  Sin : Trigonometry
  Sin1 : Trigonometry  Operator=cos
  Sum3 : Sum  Inputs=+|-
  "We " : Outport  VectorParamsAs1DForOutWhenUnconnected=off
  theta : Outport  Port=2  VectorParamsAs1DForOutWhenUnconnected=off
  wires:
  Sum3/1 -> Discrete PID Controller/1
  Product/1 -> Sum3/1
  Discrete PID Controller/1 -> "We "/1, Discrete-Time Integrator/1
  Discrete-Time Integrator/1 -> theta/1, Sin1/1, Sin/1
  Sin1/1 -> Product1/2
  Sin/1 -> Product/1
  Ialfa_h/1 -> Product/2
  Product1/1 -> Sum3/2
  "Ibeta_h "/1 -> Product1/1

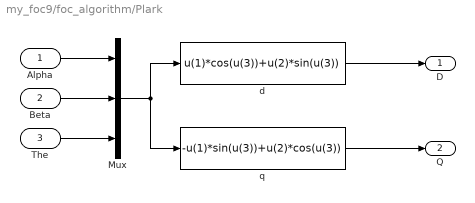
== system my_foc9/foc_algorithm/Plark ==
  Alpha : Inport
  Beta : Inport  Port=2
  The : Inport  Port=3
  Mux : Mux  Inputs=3
  d : Fcn  Expr=u(1)*cos(u(3))+u(2)*sin(u(3))
  q : Fcn  Expr=-u(1)*sin(u(3))+u(2)*cos(u(3))
  D : Outport  VectorParamsAs1DForOutWhenUnconnected=off
  Q : Outport  Port=2  VectorParamsAs1DForOutWhenUnconnected=off
  wires:
  d/1 -> D/1
  Beta/1 -> Mux/2
  The/1 -> Mux/3
  Alpha/1 -> Mux/1
  Mux/1 -> q/1, d/1
  q/1 -> Q/1

== system my_foc9/foc_algorithm/Subsystem ==
  "err " : Inport
  Discrete-Time Integrator : DiscreteIntegrator  InitialCondition=init  SampleTime=TS  LimitOutput=on  UpperSaturationLimit=Intergral_upper  LowerSaturationLimit=Intergral_lower  ICPrevOutput=DiscIntNeverNeededParam  ICPrevScaledInput=DiscIntNeverNeededParam
  Gain : Gain  Gain=kp
  Gain1 : Gain  Gain=ki
  Saturation : Saturate  UpperLimit=Out_upper  LowerLimit=Out_lower
  Subtract : Sum
  Zero-Order Hold : ZeroOrderHold  SampleTime=TS
  Out1 : Outport  VectorParamsAs1DForOutWhenUnconnected=off
  wires:
  Subtract/1 -> Saturation/1
  Gain/1 -> Zero-Order Hold/1
  Saturation/1 -> Out1/1
  Zero-Order Hold/1 -> Subtract/1
  "err "/1 -> Gain1/1, Gain/1
  Gain1/1 -> Discrete-Time Integrator/1
  Discrete-Time Integrator/1 -> Subtract/2

== system my_foc9/foc_algorithm/Subsystem1 ==
  "err " : Inport
  Discrete-Time Integrator : DiscreteIntegrator  InitialCondition=init  SampleTime=TS  LimitOutput=on  UpperSaturationLimit=Intergral_upper  LowerSaturationLimit=Intergral_lower  ICPrevOutput=DiscIntNeverNeededParam  ICPrevScaledInput=DiscIntNeverNeededParam
  Gain : Gain  Gain=kp
  Gain1 : Gain  Gain=ki
  Saturation : Saturate  UpperLimit=Out_upper  LowerLimit=Out_lower
  Subtract : Sum
  Zero-Order Hold : ZeroOrderHold  SampleTime=TS
  Out1 : Outport  VectorParamsAs1DForOutWhenUnconnected=off
  wires:
  Discrete-Time Integrator/1 -> Subtract/2
  Gain1/1 -> Discrete-Time Integrator/1
  "err "/1 -> Gain/1, Gain1/1
  Zero-Order Hold/1 -> Subtract/1
  Saturation/1 -> Out1/1
  Gain/1 -> Zero-Order Hold/1
  Subtract/1 -> Saturation/1

== system my_foc9/foc_algorithm/N_S_direction/Subsystem2 ==
  In1 : Inport
  Trigger : TriggerPort  VariantControl=Variant  PortDimensions=1
  Out1 : Outport  VectorParamsAs1DForOutWhenUnconnected=off
  wires:
  In1/1 -> Out1/1

== matlab function my_foc9/foc_algorithm/SVPWM MATLAB Function ==
  data: Valpha input single size=1; Tcmp1 output single size=1; Vbeta input single size=1; Tcmp2 output single size=1; Tcmp3 output single size=1; Udc input single size=1; Tpwm input single size=1; sector output single size=1
function [Tcmp1,Tcmp2,Tcmp3,sector] = fcn(Valpha,Vbeta,Udc,Tpwm)
%#codegen

sector = single(0);
Tcmp1 = single(0);
Tcmp2 = single(0);
Tcmp3 = single(0);

%========Parameters statement================

    Vref1 = Vbeta;							                   
    Vref2 = (sqrt(3)*Valpha - Vbeta)/2; 				    
    Vref3 = (-sqrt(3)*Valpha - Vbeta)/2;					
   
 %========Sector calculation=================

  if (Vref1>0)
	   sector = single(1);
  end
  if (Vref2>0)
	   sector = sector+single(2);
  end
  if (Vref3>0)
       sector = sector+single(4);
  end

%======== X Y Z calculation===================

X = sqrt(3)*Vbeta*Tpwm/Udc;
Y = Tpwm/Udc*(3/2*Valpha+sqrt(3)/2*Vbeta);
Z = Tpwm/Udc*(-3/2*Valpha+sqrt(3)/2*Vbeta);	         

%==========Duty ratio calculation================
switch (sector)   
    case 1
        T1 = Z; T2 = Y; 
	case 2
        T1 = Y; T2 = -X; 
	case 3
        T1 = -Z; T2 = X; 
	case 4
        T1 = -X; T2 = Z;
	case 5
        T1 = X; T2 = -Y;
    otherwise
        T1 = -Y; T2 = -Z;
end

if T1+T2 > Tpwm
    T1 = T1/(T1+T2);
    T2 = T2/(T1+T2);
else
    T1 = T1;
    T2 = T2;
end
ta = (Tpwm-(T1+T2))/4.0;
tb = ta+T1/2;
tc = tb+T2/2;

%==========Duty ratio calculation================
switch (sector)
    case 1 
        Tcmp1=tb;
        Tcmp2=ta;
        Tcmp3=tc; 
        
    case 2 
        Tcmp1=ta;
        Tcmp2=tc;
        Tcmp3=tb; 
       
    case 3 
        Tcmp1=ta;
        Tcmp2=tb;
        Tcmp3=tc; 
        
    case 4 
        Tcmp1=tc;
        Tcmp2=tb;
        Tcmp3=ta;
        
    case 5 
        Tcmp1=tc;
        Tcmp2=ta;
        Tcmp3=tb;
        
   case 6
       Tcmp1=tb;
       Tcmp2=tc;
       Tcmp3=ta;
end
end
